simulink model "ES209A_CurrMeasCorrln"  (R2013b)
settings: Solver=FixedStepDiscrete  SolverMode=SingleTasking  StartTime=0.0  StopTime=1  FixedStep=0.000125  RelTol=1e-3
values from neighbouring files (symbols this model uses):
  CurrMeasCorrlnMaxErrCurr = DataDict.Calibration    [ES209A_CurrMeasCorrln_DataDict.m]
  CurrMeasCorrlnMaxStallCntr = DataDict.Calibration    [ES209A_CurrMeasCorrln_DataDict.m]
  CurrMeasCorrlnNtc0x04DFailStep = DataDict.Calibration    [ES209A_CurrMeasCorrln_DataDict.m]
  CurrMeasCorrlnNtc0x04DPassStep = DataDict.Calibration    [ES209A_CurrMeasCorrln_DataDict.m]
  CurrMeasCorrlnNtc0x04EFailStep = DataDict.Calibration    [ES209A_CurrMeasCorrln_DataDict.m]
  CurrMeasCorrlnNtc0x04EPassStep = DataDict.Calibration    [ES209A_CurrMeasCorrln_DataDict.m]
  ELECGLBPRM_IVTRCNT_CNT_U08 = DataDict.ConfigParam    [ES209A_CurrMeasCorrln_DataDict.m]
  FLTINJ_CURRMEASCORRLN_CURRMEASIDPTSIG = DataDict.Constant    [ES209A_CurrMeasCorrln_DataDict.m]
libraries: NxtrLim x2, simulink x1
(part 2 of 2)

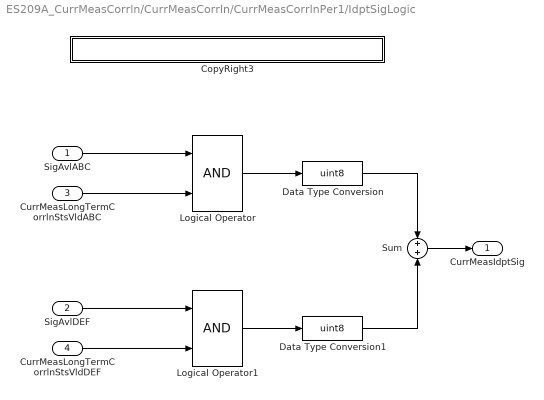
== system ES209A_CurrMeasCorrln/CurrMeasCorrln/CurrMeasCorrlnPer1/IdptSigLogic ==
  SigAvlABC : Inport  RequirementInfo={'linktype_rmi_doors' '0000c46e (/ESG Group/FDD Module Requirements/EA4 Specific/ES209A_CurrMeasCorrln)' '#ES209A_217' 'true' 'REQ: ES209A_217' '' ; 'linktype_rmi_doors' '0000c46e (/ESG Group/FDD Module Requirements/EA4 Specific/ES209A_CurrMeasCorrln)' '#ES209A_228' 'true' 'REQ: ES209A_228' '' ; 'linktype_rmi_doors' '0000c46e (/ESG Group/FDD Module Requirements/EA4 Specific/ES209A_CurrMeasCorrln)' '#ES209A_230' 'true' 'REQ: ES209A_230' '' ; 'linktype_rmi_doors' '0000c46e (/ESG Group/FDD Module Requirements/EA4 Specific/ES209A_CurrMeasCorrln)' '#ES209A_229' 'true' 'REQ: ES209A_229' '' } %GIDa_942e1c7b_ad02_468a_aa2a_044d99b82600
  SigAvlDEF : Inport  RequirementInfo={'linktype_rmi_doors' '0000c46e (/ESG Group/FDD Module Requirements/EA4 Specific/ES209A_CurrMeasCorrln)' '#ES209A_217' 'true' 'REQ: ES209A_217' '' ; 'linktype_rmi_doors' '0000c46e (/ESG Group/FDD Module Requirements/EA4 Specific/ES209A_CurrMeasCorrln)' '#ES209A_228' 'true' 'REQ: ES209A_228' '' ; 'linktype_rmi_doors' '0000c46e (/ESG Group/FDD Module Requirements/EA4 Specific/ES209A_CurrMeasCorrln)' '#ES209A_230' 'true' 'REQ: ES209A_230' '' ; 'linktype_rmi_doors' '0000c46e (/ESG Group/FDD Module Requirements/EA4 Specific/ES209A_CurrMeasCorrln)' '#ES209A_229' 'true' 'REQ: ES209A_229' '' } %GIDa_d76c2ed2_628a_4e52_8d10_5cc2fe66b57a  Port=2
  CurrMeasLongTermCorrlnStsVldABC : Inport  RequirementInfo={'linktype_rmi_doors' '0000c46e (/ESG Group/FDD Module Requirements/EA4 Specific/ES209A_CurrMeasCorrln)' '#ES209A_217' 'true' 'REQ: ES209A_217' '' ; 'linktype_rmi_doors' '0000c46e (/ESG Group/FDD Module Requirements/EA4 Specific/ES209A_CurrMeasCorrln)' '#ES209A_228' 'true' 'REQ: ES209A_228' '' ; 'linktype_rmi_doors' '0000c46e (/ESG Group/FDD Module Requirements/EA4 Specific/ES209A_CurrMeasCorrln)' '#ES209A_230' 'true' 'REQ: ES209A_230' '' ; 'linktype_rmi_doors' '0000c46e (/ESG Group/FDD Module Requirements/EA4 Specific/ES209A_CurrMeasCorrln)' '#ES209A_229' 'true' 'REQ: ES209A_229' '' } %GIDa_55133441_4ac9_4891_99c3_8d3056d5d792  Port=3
  CurrMeasLongTermCorrlnStsVldDEF : Inport  RequirementInfo={'linktype_rmi_doors' '0000c46e (/ESG Group/FDD Module Requirements/EA4 Specific/ES209A_CurrMeasCorrln)' '#ES209A_217' 'true' 'REQ: ES209A_217' '' ; 'linktype_rmi_doors' '0000c46e (/ESG Group/FDD Module Requirements/EA4 Specific/ES209A_CurrMeasCorrln)' '#ES209A_228' 'true' 'REQ: ES209A_228' '' ; 'linktype_rmi_doors' '0000c46e (/ESG Group/FDD Module Requirements/EA4 Specific/ES209A_CurrMeasCorrln)' '#ES209A_230' 'true' 'REQ: ES209A_230' '' ; 'linktype_rmi_doors' '0000c46e (/ESG Group/FDD Module Requirements/EA4 Specific/ES209A_CurrMeasCorrln)' '#ES209A_229' 'true' 'REQ: ES209A_229' '' } %GIDa_bf3bd0c8_6e6b_4ddf_a539_8fba819f64a3  Port=4
  CopyRight3 : Subsystem  Description=|  mask(Copyright Information){none=on}
      | Copyright info block.                                               
      |                                                                     
      | Place copyright information at the top of every subsystem in design.
      mask prompts: none "No parameters"
      mask help: Place copyright information at the top of every subsystem in design.
      mask Display:
      | NxtrConf = 'Nexteer Confidential';
      | 
      | sys = bdroot; %handle for the current model ("system")
      | first = get_param(sys,'Created');
      | first = first(end-3:end);  %year is last four digits
      | 
      | last = get_param(sys,'LastModifiedDate');
      | if isempty(last)
      |     last = datestr(now,'yyyy');
      | else
      |     last = last(end-3:end);
      | end
      | 
      | if strcmp(first,last)
      |     fprintf('%s -- Copyright %s Nexteer',NxtrConf,first)
      | else
      |     fprintf('%s -- %s%s- %s Nexteer',NxtrConf,char(169),first,last)
      | end
  Data Type Conversion : DataTypeConversion  RequirementInfo={'linktype_rmi_doors' '0000c46e (/ESG Group/FDD Module Requirements/EA4 Specific/ES209A_CurrMeasCorrln)' '#ES209A_217' 'true' 'REQ: ES209A_217' '' ; 'linktype_rmi_doors' '0000c46e (/ESG Group/FDD Module Requirements/EA4 Specific/ES209A_CurrMeasCorrln)' '#ES209A_228' 'true' 'REQ: ES209A_228' '' ; 'linktype_rmi_doors' '0000c46e (/ESG Group/FDD Module Requirements/EA4 Specific/ES209A_CurrMeasCorrln)' '#ES209A_230' 'true' 'REQ: ES209A_230' '' ; 'linktype_rmi_doors' '0000c46e (/ESG Group/FDD Module Requirements/EA4 Specific/ES209A_CurrMeasCorrln)' '#ES209A_229' 'true' 'REQ: ES209A_229' '' } %GIDa_5ccb0532_ac29_46e4_aa67_eafed2953408  OutDataTypeStr=uint8
  Data Type Conversion1 : DataTypeConversion  RequirementInfo={'linktype_rmi_doors' '0000c46e (/ESG Group/FDD Module Requirements/EA4 Specific/ES209A_CurrMeasCorrln)' '#ES209A_217' 'true' 'REQ: ES209A_217' '' ; 'linktype_rmi_doors' '0000c46e (/ESG Group/FDD Module Requirements/EA4 Specific/ES209A_CurrMeasCorrln)' '#ES209A_228' 'true' 'REQ: ES209A_228' '' ; 'linktype_rmi_doors' '0000c46e (/ESG Group/FDD Module Requirements/EA4 Specific/ES209A_CurrMeasCorrln)' '#ES209A_230' 'true' 'REQ: ES209A_230' '' ; 'linktype_rmi_doors' '0000c46e (/ESG Group/FDD Module Requirements/EA4 Specific/ES209A_CurrMeasCorrln)' '#ES209A_229' 'true' 'REQ: ES209A_229' '' } %GIDa_14c0623b_5dcd_41aa_bf12_39046edbd1db  OutDataTypeStr=uint8
  Logical Operator : Logic  RequirementInfo={'linktype_rmi_doors' '0000c46e (/ESG Group/FDD Module Requirements/EA4 Specific/ES209A_CurrMeasCorrln)' '#ES209A_217' 'true' 'REQ: ES209A_217' '' ; 'linktype_rmi_doors' '0000c46e (/ESG Group/FDD Module Requirements/EA4 Specific/ES209A_CurrMeasCorrln)' '#ES209A_228' 'true' 'REQ: ES209A_228' '' ; 'linktype_rmi_doors' '0000c46e (/ESG Group/FDD Module Requirements/EA4 Specific/ES209A_CurrMeasCorrln)' '#ES209A_230' 'true' 'REQ: ES209A_230' '' ; 'linktype_rmi_doors' '0000c46e (/ESG Group/FDD Module Requirements/EA4 Specific/ES209A_CurrMeasCorrln)' '#ES209A_229' 'true' 'REQ: ES209A_229' '' } %GIDa_2d1d910d_56b5_4346_ba27_43432a5aa696  IconShape=distinctive  AllPortsSameDT=off  OutDataTypeStr=boolean
  Logical Operator1 : Logic  RequirementInfo={'linktype_rmi_doors' '0000c46e (/ESG Group/FDD Module Requirements/EA4 Specific/ES209A_CurrMeasCorrln)' '#ES209A_217' 'true' 'REQ: ES209A_217' '' ; 'linktype_rmi_doors' '0000c46e (/ESG Group/FDD Module Requirements/EA4 Specific/ES209A_CurrMeasCorrln)' '#ES209A_228' 'true' 'REQ: ES209A_228' '' ; 'linktype_rmi_doors' '0000c46e (/ESG Group/FDD Module Requirements/EA4 Specific/ES209A_CurrMeasCorrln)' '#ES209A_230' 'true' 'REQ: ES209A_230' '' ; 'linktype_rmi_doors' '0000c46e (/ESG Group/FDD Module Requirements/EA4 Specific/ES209A_CurrMeasCorrln)' '#ES209A_229' 'true' 'REQ: ES209A_229' '' } %GIDa_f9654050_ad02_4c8d_9892_cac1300cf1d7  IconShape=distinctive  AllPortsSameDT=off  OutDataTypeStr=boolean
  Sum : Sum  RequirementInfo={'linktype_rmi_doors' '0000c46e (/ESG Group/FDD Module Requirements/EA4 Specific/ES209A_CurrMeasCorrln)' '#ES209A_217' 'true' 'REQ: ES209A_217' '' ; 'linktype_rmi_doors' '0000c46e (/ESG Group/FDD Module Requirements/EA4 Specific/ES209A_CurrMeasCorrln)' '#ES209A_228' 'true' 'REQ: ES209A_228' '' ; 'linktype_rmi_doors' '0000c46e (/ESG Group/FDD Module Requirements/EA4 Specific/ES209A_CurrMeasCorrln)' '#ES209A_230' 'true' 'REQ: ES209A_230' '' ; 'linktype_rmi_doors' '0000c46e (/ESG Group/FDD Module Requirements/EA4 Specific/ES209A_CurrMeasCorrln)' '#ES209A_229' 'true' 'REQ: ES209A_229' '' } %GIDa_4ade3bee_f5e6_4a94_82c8_89a81567cdbe  Inputs=+|+
  CurrMeasIdptSig : Outport  RequirementInfo={'linktype_rmi_doors' '0000c46e (/ESG Group/FDD Module Requirements/EA4 Specific/ES209A_CurrMeasCorrln)' '#ES209A_217' 'true' 'REQ: ES209A_217' '' ; 'linktype_rmi_doors' '0000c46e (/ESG Group/FDD Module Requirements/EA4 Specific/ES209A_CurrMeasCorrln)' '#ES209A_228' 'true' 'REQ: ES209A_228' '' ; 'linktype_rmi_doors' '0000c46e (/ESG Group/FDD Module Requirements/EA4 Specific/ES209A_CurrMeasCorrln)' '#ES209A_230' 'true' 'REQ: ES209A_230' '' ; 'linktype_rmi_doors' '0000c46e (/ESG Group/FDD Module Requirements/EA4 Specific/ES209A_CurrMeasCorrln)' '#ES209A_229' 'true' 'REQ: ES209A_229' '' } %GIDa_242059a7_1f05_43ee_b251_027ca547b730
  wires:
  SigAvlABC/1 -> Logical Operator/1
  CurrMeasLongTermCorrlnStsVldABC/1 -> Logical Operator/2
  CurrMeasLongTermCorrlnStsVldDEF/1 -> Logical Operator1/2
  SigAvlDEF/1 -> Logical Operator1/1
  Logical Operator/1 -> Data Type Conversion/1
  Logical Operator1/1 -> Data Type Conversion1/1
  Data Type Conversion/1 -> Sum/1
  Data Type Conversion1/1 -> Sum/2
  Sum/1 -> CurrMeasIdptSig/1

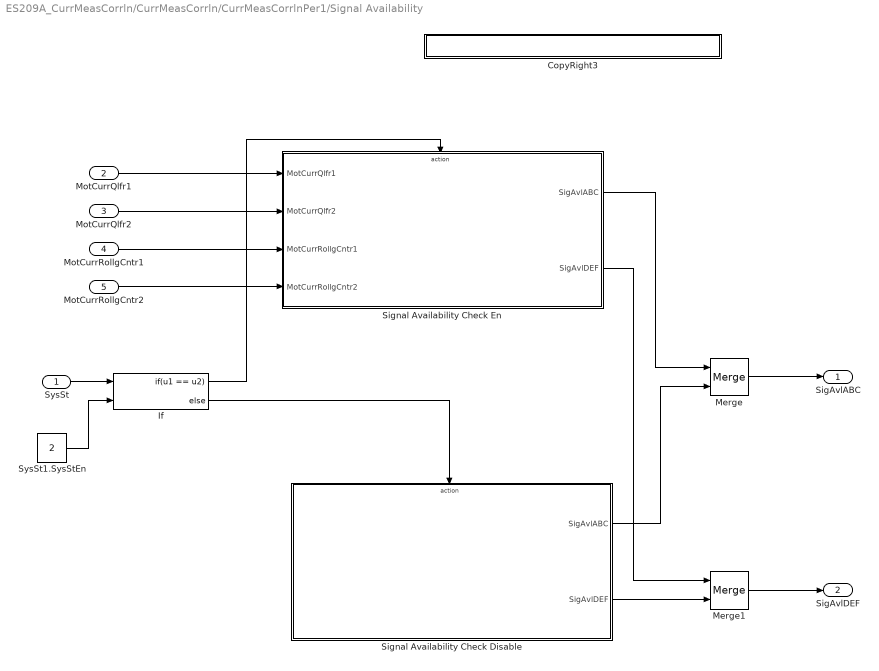
== system ES209A_CurrMeasCorrln/CurrMeasCorrln/CurrMeasCorrlnPer1/Signal Availability ==
  SysSt : Inport  RequirementInfo={} %GIDa_1186099d_dc67_4f7c_b378_ee59f8c97963  OutDataTypeStr=uint8
  MotCurrQlfr1 : Inport  RequirementInfo={} %GIDa_9546d9ec_22e7_463e_bbd0_54a2b6352662  Port=2
  MotCurrQlfr2 : Inport  RequirementInfo={} %GIDa_d3dc025e_ce3e_43df_848d_21e84192c51e  Port=3
  MotCurrRollgCntr1 : Inport  RequirementInfo={} %GIDa_8e4ee91b_32ff_41c2_995e_2ae76632680d  Port=4
  MotCurrRollgCntr2 : Inport  RequirementInfo={} %GIDa_46b1cb0c_dece_4346_b2ac_908178a65c66  Port=5
  CopyRight3 : Subsystem  Description=|  mask(Copyright Information){none=on}
      | Copyright info block.                                               
      |                                                                     
      | Place copyright information at the top of every subsystem in design.
      mask prompts: none "No parameters"
      mask help: Place copyright information at the top of every subsystem in design.
      mask Display:
      | NxtrConf = 'Nexteer Confidential';
      | 
      | sys = bdroot; %handle for the current model ("system")
      | first = get_param(sys,'Created');
      | first = first(end-3:end);  %year is last four digits
      | 
      | last = get_param(sys,'LastModifiedDate');
      | if isempty(last)
      |     last = datestr(now,'yyyy');
      | else
      |     last = last(end-3:end);
      | end
      | 
      | if strcmp(first,last)
      |     fprintf('%s -- Copyright %s Nexteer',NxtrConf,first)
      | else
      |     fprintf('%s -- %s%s- %s Nexteer',NxtrConf,char(169),first,last)
      | end
  If : If  NumInputs=2  IfExpression=u1 == u2
  Merge : Merge
  Merge1 : Merge
  Signal Availability Check Disable : Subsystem  RequirementInfo={} %GIDa_6318f0e3_a9ed_4028_939a_acdca8fc9a22  TreatAsAtomicUnit=on
  Signal Availability Check En : Subsystem  RequirementInfo={'linktype_rmi_doors' '0000c46e (/ESG Group/FDD Module Requirements/EA4 Specific/ES209A CurrMeasCorrln)' '#ES209A_135' 'true' 'REQ: ES209A_135' '' } %GIDa_7e57cf61_2110_43cd_98fc_69fb451c1a76  TreatAsAtomicUnit=on
  SysSt1.SysStEn : Constant  Value=2  OutDataTypeStr=uint8
  SigAvlABC : Outport
  SigAvlDEF : Outport  Port=2
  wires:
  SysSt/1 -> If/1
  SysSt1.SysStEn/1 -> If/2
  MotCurrQlfr1/1 -> Signal Availability Check En/1(MotCurrQlfr1)
  MotCurrQlfr2/1 -> Signal Availability Check En/2(MotCurrQlfr2)
  MotCurrRollgCntr1/1 -> Signal Availability Check En/3(MotCurrRollgCntr1)
  MotCurrRollgCntr2/1 -> Signal Availability Check En/4(MotCurrRollgCntr2)
  Signal Availability Check En/1(SigAvlABC) -> Merge/1
  Signal Availability Check Disable/1(SigAvlABC) -> Merge/2
  Signal Availability Check En/2("SigAvlDEF ") -> Merge1/1
  Signal Availability Check Disable/2("SigAvlDEF ") -> Merge1/2
  Merge/1 -> SigAvlABC/1
  Merge1/1 -> SigAvlDEF/1
  If/2 -> Signal Availability Check Disable/Action
  If/1 -> Signal Availability Check En/Action

== system ES209A_CurrMeasCorrln/CurrMeasCorrln/CurrMeasCorrlnPer1/CorrlnChkABC/GetNtcQlfrSts/CopyRight2 ==

== system ES209A_CurrMeasCorrln/CurrMeasCorrln/CurrMeasCorrlnPer1/CorrlnChkABC/ImdtCorrlnCk/CopyRight2 ==

== system ES209A_CurrMeasCorrln/CurrMeasCorrln/CurrMeasCorrlnPer1/CorrlnChkABC/ImdtCorrlnCk/If Action Subsystem ==
  Action Port : ActionPort  ActionType=then
  Constant : Constant
  ImdtCorrlnABC : Outport
  wires:
  Constant/1 -> ImdtCorrlnABC/1

== system ES209A_CurrMeasCorrln/CurrMeasCorrln/CurrMeasCorrlnPer1/CorrlnChkABC/ImdtCorrlnCk/If Action Subsystem1 ==
  Action Port : ActionPort  ActionType=else
  Constant : Constant  Value=0
  ImdtCorrlnABC : Outport
  wires:
  Constant/1 -> ImdtCorrlnABC/1

== system ES209A_CurrMeasCorrln/CurrMeasCorrln/CurrMeasCorrlnPer1/CorrlnChkABC/SetNtcSts/CopyRight2 ==

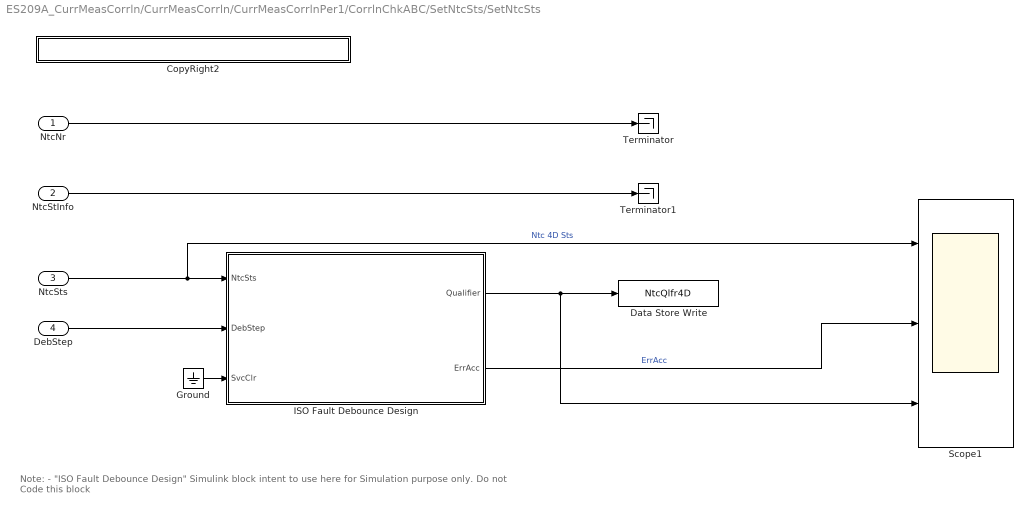
== system ES209A_CurrMeasCorrln/CurrMeasCorrln/CurrMeasCorrlnPer1/CorrlnChkABC/SetNtcSts/SetNtcSts ==
  note: Note:
      |
      | - "ISO Fault Debounce Design" Simulink block intent to use here for Simulation purpose only. Do not Code this block
  NtcNr : Inport
  NtcStInfo : Inport  Port=2
  NtcSts : Inport  Port=3
  DebStep : Inport  Port=4
  CopyRight2 : Subsystem  Description=|  mask(Copyright Information){none=on}
      | Copyright info block.                                               
      |                                                                     
      | Place copyright information at the top of every subsystem in design.
      mask prompts: none "No parameters"
      mask help: Place copyright information at the top of every subsystem in design.
      mask Display:
      | NxtrConf = 'Nexteer Confidential';
      | 
      | sys = bdroot; %handle for the current model ("system")
      | first = get_param(sys,'Created');
      | first = first(end-3:end);  %year is last four digits
      | 
      | last = get_param(sys,'LastModifiedDate');
      | if isempty(last)
      |     last = datestr(now,'yyyy');
      | else
      |     last = last(end-3:end);
      | end
      | 
      | if strcmp(first,last)
      |     fprintf('%s -- Copyright %s Nexteer',NxtrConf,first)
      | else
      |     fprintf('%s -- %s%s- %s Nexteer',NxtrConf,char(169),first,last)
      | end
  Data Store Write : DataStoreWrite  DataStoreName=NtcQlfr4D
  Ground : Ground
  ISO Fault Debounce Design : Stateflow chart  RequirementInfo={'linktype_rmi_doors' '0000c46e (/ESG Group/FDD Module Requirements/EA4 Specific/ES209A CurrMeasCorrln)' '#ES209A_236' 'true' 'REQ: ES209A_236' '' } %GIDa_d30caf31_34ad_4c46_80cc_2f0c0a5a5e0e  TreatAsAtomicUnit=on
      settings: AttributesFormatString=|
      | Simulation Purpose Only.
      | Do Not Code this block
      | Diagnostic Manager Owns this requirement
  Scope1 : Scope  NumInputPorts=3
      settings: YMin=2~-35000~0  YMax=3~35000~1  SaveName=ScopeData4
  Terminator : Terminator
  Terminator1 : Terminator
  wires:
  NtcStInfo/1 -> Terminator1/1
  NtcNr/1 -> Terminator/1
  DebStep/1 -> ISO Fault Debounce Design/2(DebStep)
  ISO Fault Debounce Design/1(Qualifier) -> Scope1/3, Data Store Write/1
  Ground/1 -> ISO Fault Debounce Design/3(SvcClr)
  ISO Fault Debounce Design/2(ErrAcc) -> Scope1/2  "ErrAcc"
  NtcSts/1 -> Scope1/1, ISO Fault Debounce Design/1(NtcSts)  "Ntc 4D Sts"

== system ES209A_CurrMeasCorrln/CurrMeasCorrln/CurrMeasCorrlnPer1/CorrlnChkDEF/GetNtcQlfrSts/CopyRight2 ==

== system ES209A_CurrMeasCorrln/CurrMeasCorrln/CurrMeasCorrlnPer1/CorrlnChkDEF/ImdtCorrlnCk/CopyRight2 ==

== system ES209A_CurrMeasCorrln/CurrMeasCorrln/CurrMeasCorrlnPer1/CorrlnChkDEF/ImdtCorrlnCk/If Action Subsystem ==
  Action Port : ActionPort  ActionType=then
  Constant : Constant
  ImdtCorrlnABC : Outport
  wires:
  Constant/1 -> ImdtCorrlnABC/1

== system ES209A_CurrMeasCorrln/CurrMeasCorrln/CurrMeasCorrlnPer1/CorrlnChkDEF/ImdtCorrlnCk/If Action Subsystem1 ==
  Action Port : ActionPort  ActionType=else
  Constant : Constant  Value=0
  ImdtCorrlnABC : Outport
  wires:
  Constant/1 -> ImdtCorrlnABC/1

== system ES209A_CurrMeasCorrln/CurrMeasCorrln/CurrMeasCorrlnPer1/CorrlnChkDEF/SetNtcSts/CopyRight2 ==

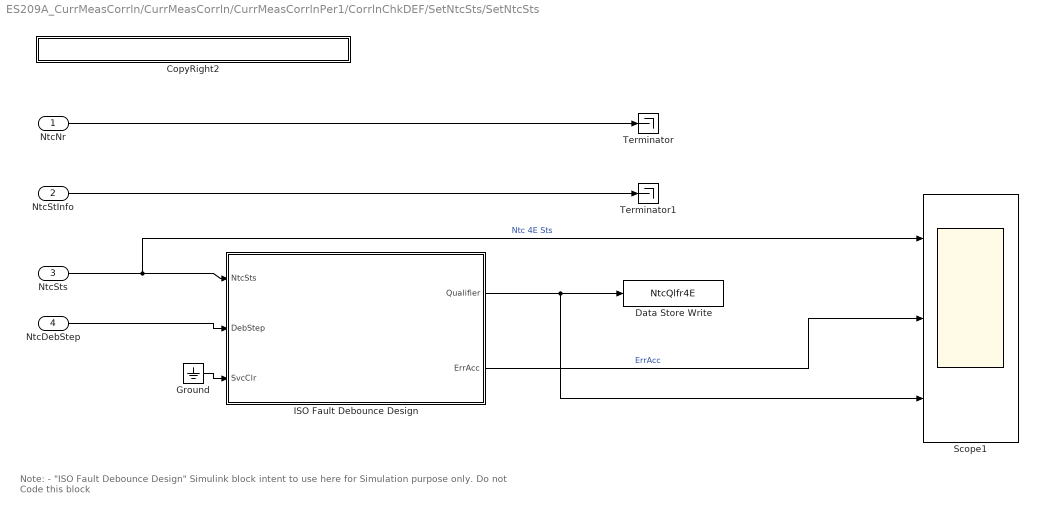
== system ES209A_CurrMeasCorrln/CurrMeasCorrln/CurrMeasCorrlnPer1/CorrlnChkDEF/SetNtcSts/SetNtcSts ==
  note: Note:
      |
      | - "ISO Fault Debounce Design" Simulink block intent to use here for Simulation purpose only. Do not Code this block
  NtcNr : Inport
  NtcStInfo : Inport  Port=2
  NtcSts : Inport  Port=3
  NtcDebStep : Inport  Port=4
  CopyRight2 : Subsystem  Description=|  mask(Copyright Information){none=on}
      | Copyright info block.                                               
      |                                                                     
      | Place copyright information at the top of every subsystem in design.
      mask prompts: none "No parameters"
      mask help: Place copyright information at the top of every subsystem in design.
      mask Display:
      | NxtrConf = 'Nexteer Confidential';
      | 
      | sys = bdroot; %handle for the current model ("system")
      | first = get_param(sys,'Created');
      | first = first(end-3:end);  %year is last four digits
      | 
      | last = get_param(sys,'LastModifiedDate');
      | if isempty(last)
      |     last = datestr(now,'yyyy');
      | else
      |     last = last(end-3:end);
      | end
      | 
      | if strcmp(first,last)
      |     fprintf('%s -- Copyright %s Nexteer',NxtrConf,first)
      | else
      |     fprintf('%s -- %s%s- %s Nexteer',NxtrConf,char(169),first,last)
      | end
  Data Store Write : DataStoreWrite  DataStoreName=NtcQlfr4E
  Ground : Ground
  ISO Fault Debounce Design : Stateflow chart  RequirementInfo={'linktype_rmi_doors' '0000c46e (/ESG Group/FDD Module Requirements/EA4 Specific/ES209A CurrMeasCorrln)' '#ES209A_252' 'true' 'REQ: ES209A_252' '' } %GIDa_7a5c8c14_f745_4195_88a1_5e88b55f3450  TreatAsAtomicUnit=on
      settings: AttributesFormatString=|
      | Simulation Purpose Only.
      | Do Not Code this block
      | Diagnostic Manager Owns this requirement
  Scope1 : Scope  NumInputPorts=3
      settings: YMin=2~-35000~0  YMax=3~35000~2  SaveName=ScopeData4
  Terminator : Terminator
  Terminator1 : Terminator
  wires:
  NtcStInfo/1 -> Terminator1/1
  NtcNr/1 -> Terminator/1
  NtcSts/1 -> ISO Fault Debounce Design/1(NtcSts), Scope1/1  "Ntc 4E Sts"
  NtcDebStep/1 -> ISO Fault Debounce Design/2(DebStep)
  ISO Fault Debounce Design/1(Qualifier) -> Scope1/3, Data Store Write/1
  Ground/1 -> ISO Fault Debounce Design/3(SvcClr)
  ISO Fault Debounce Design/2(ErrAcc) -> Scope1/2  "ErrAcc"

== system ES209A_CurrMeasCorrln/CurrMeasCorrln/CurrMeasCorrlnPer1/CorrlnStsLogic/CopyRight3 ==

== system ES209A_CurrMeasCorrln/CurrMeasCorrln/CurrMeasCorrlnPer1/FltInj_u08/CopyRight1 ==

== system ES209A_CurrMeasCorrln/CurrMeasCorrln/CurrMeasCorrlnPer1/IdptSigLogic/CopyRight3 ==

== system ES209A_CurrMeasCorrln/CurrMeasCorrln/CurrMeasCorrlnPer1/Signal Availability/CopyRight3 ==

== system ES209A_CurrMeasCorrln/CurrMeasCorrln/CurrMeasCorrlnPer1/Signal Availability/Signal Availability Check Disable ==
  Action Port : ActionPort  ActionType=else
  Constant : Constant  OutDataTypeStr=uint8
  Constant1 : Constant  OutDataTypeStr=uint8
  CopyRight3 : Subsystem  Description=|  mask(Copyright Information){none=on}
      | Copyright info block.                                               
      |                                                                     
      | Place copyright information at the top of every subsystem in design.
      mask prompts: none "No parameters"
      mask help: Place copyright information at the top of every subsystem in design.
      mask Display:
      | NxtrConf = 'Nexteer Confidential';
      | 
      | sys = bdroot; %handle for the current model ("system")
      | first = get_param(sys,'Created');
      | first = first(end-3:end);  %year is last four digits
      | 
      | last = get_param(sys,'LastModifiedDate');
      | if isempty(last)
      |     last = datestr(now,'yyyy');
      | else
      |     last = last(end-3:end);
      | end
      | 
      | if strcmp(first,last)
      |     fprintf('%s -- Copyright %s Nexteer',NxtrConf,first)
      | else
      |     fprintf('%s -- %s%s- %s Nexteer',NxtrConf,char(169),first,last)
      | end
  SigAvlABC : Outport
  "SigAvlDEF " : Outport  Port=2
  wires:
  Constant1/1 -> "SigAvlDEF "/1
  Constant/1 -> SigAvlABC/1

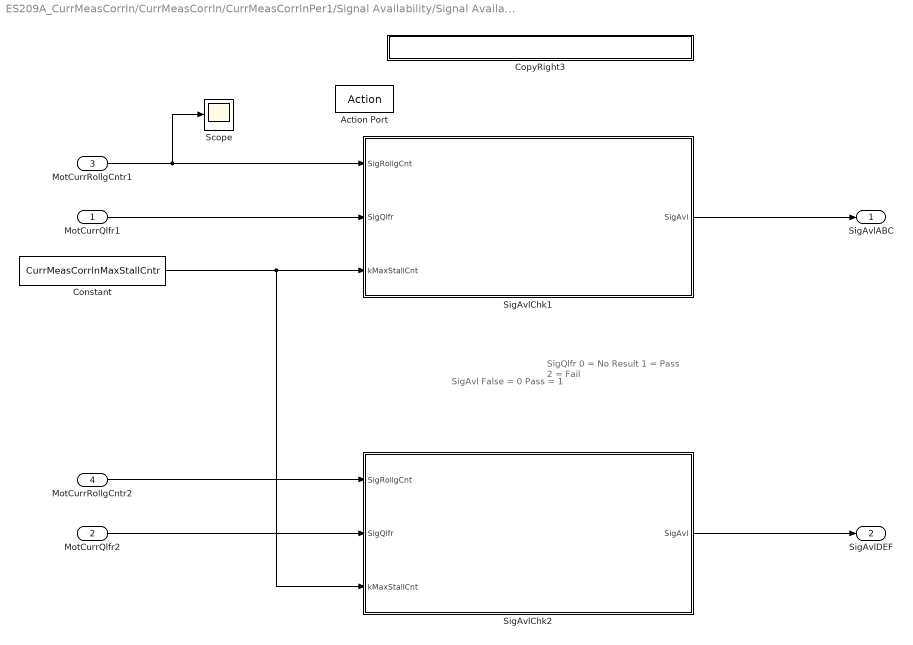
== system ES209A_CurrMeasCorrln/CurrMeasCorrln/CurrMeasCorrlnPer1/Signal Availability/Signal Availability Check En ==
  note: SigQlfr
      | 0 = No Result
      | 1 = Pass
      | 2 = Fail
  note: SigAvl
      | False = 0
      | Pass = 1
  MotCurrQlfr1 : Inport  RequirementInfo={} %GIDa_023689e3_7c9e_4df1_83a1_699197148238
  MotCurrQlfr2 : Inport  RequirementInfo={} %GIDa_7e6e4398_831d_4c26_91b8_cbf4c078805f  Port=2
  MotCurrRollgCntr1 : Inport  RequirementInfo={} %GIDa_382efb02_9c14_4780_8bc5_4a8377343de5  Port=3
  MotCurrRollgCntr2 : Inport  RequirementInfo={} %GIDa_533c6f48_88f4_4233_bfc1_2f844aa0d431  Port=4
  Action Port : ActionPort  ActionType=then
  Constant : Constant  Value=CurrMeasCorrlnMaxStallCntr
  CopyRight3 : Subsystem  Description=|  mask(Copyright Information){none=on}
      | Copyright info block.                                               
      |                                                                     
      | Place copyright information at the top of every subsystem in design.
      mask prompts: none "No parameters"
      mask help: Place copyright information at the top of every subsystem in design.
      mask Display:
      | NxtrConf = 'Nexteer Confidential';
      | 
      | sys = bdroot; %handle for the current model ("system")
      | first = get_param(sys,'Created');
      | first = first(end-3:end);  %year is last four digits
      | 
      | last = get_param(sys,'LastModifiedDate');
      | if isempty(last)
      |     last = datestr(now,'yyyy');
      | else
      |     last = last(end-3:end);
      | end
      | 
      | if strcmp(first,last)
      |     fprintf('%s -- Copyright %s Nexteer',NxtrConf,first)
      | else
      |     fprintf('%s -- %s%s- %s Nexteer',NxtrConf,char(169),first,last)
      | end
  Scope : Scope
  SigAvlChk1 : Subsystem  RequirementInfo={'linktype_rmi_doors' '0000c46e (/ESG Group/FDD Module Requirements/EA4 Specific/ES209A CurrMeasCorrln)' '#ES209A_135' 'true' 'REQ: ES209A_135' '' } %GIDa_5a6e0e53_d246_4b66_936c_563396a92aca  TreatAsAtomicUnit=on
  SigAvlChk2 : Subsystem  RequirementInfo={'linktype_rmi_doors' '0000c46e (/ESG Group/FDD Module Requirements/EA4 Specific/ES209A CurrMeasCorrln)' '#ES209A_219' 'true' 'REQ: ES209A_219' '' } %GIDa_e73a73aa_ed9a_4202_a7ed_28e935db4abc  TreatAsAtomicUnit=on
  SigAvlABC : Outport
  "SigAvlDEF " : Outport  Port=2
  wires:
  MotCurrRollgCntr1/1 -> SigAvlChk1/1(SigRollgCnt), Scope/1
  MotCurrQlfr1/1 -> SigAvlChk1/2(SigQlfr)
  MotCurrRollgCntr2/1 -> SigAvlChk2/1(SigRollgCnt)
  MotCurrQlfr2/1 -> SigAvlChk2/2(SigQlfr)
  Constant/1 -> SigAvlChk2/3(kMaxStallCnt), SigAvlChk1/3(kMaxStallCnt)
  SigAvlChk2/1(SigAvl) -> "SigAvlDEF "/1
  SigAvlChk1/1(SigAvl) -> SigAvlABC/1

== system ES209A_CurrMeasCorrln/CurrMeasCorrln/CurrMeasCorrlnPer1/CorrlnChkABC/SetNtcSts/SetNtcSts/CopyRight2 ==

== system ES209A_CurrMeasCorrln/CurrMeasCorrln/CurrMeasCorrlnPer1/CorrlnChkDEF/SetNtcSts/SetNtcSts/CopyRight2 ==

== system ES209A_CurrMeasCorrln/CurrMeasCorrln/CurrMeasCorrlnPer1/Signal Availability/Signal Availability Check Disable/CopyRight3 ==

== system ES209A_CurrMeasCorrln/CurrMeasCorrln/CurrMeasCorrlnPer1/Signal Availability/Signal Availability Check En/CopyRight3 ==

== system ES209A_CurrMeasCorrln/CurrMeasCorrln/CurrMeasCorrlnPer1/Signal Availability/Signal Availability Check En/SigAvlChk1 ==
  note: Example of PIM declaration for StallCnt State Variable
      |
      | SnsrShoNameSens0StallCntPrev = DataDict.PIM;
      | SnsrShoNameSens0StallCntPrev.LongName = 'SnsrShoNameSens0RollgCntPrev';
      | SnsrShoNameSens0StallCntPrev.Description = 'SnsrShoNameSens0RollgCntPrev';
      | SnsrShoNameSens0StallCntPrev.DocUnits = 'Cnt';
      | SnsrShoNameSens0StallCntPrev.EngDT = dt.u08;
      | SnsrShoNameSens0StallCntPrev.EngInit = 0;
      | SnsrShoNameSens0StallCntPrev.EngMin = 0;
      | SnsrShoNameSens0StallCntPrev.EngMax = 255;
      |
      |
      | *********  Need different state variable for each instance of this  subsystem ********
  note: Example of PIM declaration for RollgCnt State Variable
      |
      | SnsrShoNameSens0RollgCntPrev = DataDict.PIM;
      | SnsrShoNameSens0RollgCntPrev.LongName = 'SnsrShoNameSens0RollgCntPrev';
      | SnsrShoNameSens0RollgCntPrev.Description = 'SnsrShoNameSens0RollgCntPrev';
      | SnsrShoNameSens0RollgCntPrev.DocUnits = 'Cnt';
      | SnsrShoNameSens0RollgCntPrev.EngDT = dt.u08;
      | SnsrShoNameSens0RollgCntPrev.EngInit = 0;
      | SnsrShoNameSens0RollgCntPrev.EngMin = 0;
      | SnsrShoNameSens0RollgCntPrev.EngMax = 255;
      |
      |
      | *********  Need different state variable for each instance of this  subsystem ********
  SigRollgCnt : Inport  OutDataTypeStr=uint8
  SigQlfr : Inport  Port=2  OutDataTypeStr=uint8
  kMaxStallCnt : Inport  Port=3  OutDataTypeStr=uint8
  CopyRight1 : Subsystem  Description=|  mask(Copyright Information){none=on}
      | Copyright info block.                                               
      |                                                                     
      | Place copyright information at the top of every subsystem in design.
      mask prompts: none "No parameters"
      mask help: Place copyright information at the top of every subsystem in design.
      mask Display:
      | NxtrConf = 'Nexteer Confidential';
      | 
      | sys = bdroot; %handle for the current model ("system")
      | first = get_param(sys,'Created');
      | first = first(end-3:end);  %year is last four digits
      | 
      | last = get_param(sys,'LastModifiedDate');
      | if isempty(last)
      |     last = datestr(now,'yyyy');
      | else
      |     last = last(end-3:end);
      | end
      | 
      | if strcmp(first,last)
      |     fprintf('%s -- Copyright %s Nexteer',NxtrConf,first)
      | else
      |     fprintf('%s -- %s%s- %s Nexteer',NxtrConf,char(169),first,last)
      | end
  Display2 : Display
  Display3 : Display
  SigAvlChkRev2 : Stateflow chart  TreatAsAtomicUnit=on
  Unit Delay : UnitDelay  SampleTime=-1  StateName=Snsr0RollgCntPrev  StateMustResolveToSignalObject=on
      settings: AttributesFormatString=|
      | State Variable:
      | %<StateName>
  Unit Delay1 : UnitDelay  SampleTime=-1  StateName=Snsr0StallCntPrev  StateMustResolveToSignalObject=on
      settings: AttributesFormatString=|
      | State Variable:
      | %<StateName>
  SigAvl : Outport
  wires:
  SigRollgCnt/1 -> Unit Delay/1, Display2/1, SigAvlChkRev2/1(SigRollgCnt)  "SigRollgCnt"
  SigQlfr/1 -> Display3/1, SigAvlChkRev2/2(SigQlfr)  "SigQlfr"
  kMaxStallCnt/1 -> SigAvlChkRev2/3(kMaxStallCnt)  "kMaxStallCnt"
  Unit Delay/1 -> SigAvlChkRev2/4(LstRollgCnt)
  SigAvlChkRev2/2(StallCntOutp) -> Unit Delay1/1
  Unit Delay1/1 -> SigAvlChkRev2/5(LstStallCnt)
  SigAvlChkRev2/1(SigAvl) -> SigAvl/1

== system ES209A_CurrMeasCorrln/CurrMeasCorrln/CurrMeasCorrlnPer1/Signal Availability/Signal Availability Check En/SigAvlChk2 ==
  note: Example of PIM declaration for StallCnt State Variable
      |
      | SnsrShoNameSens0StallCntPrev = DataDict.PIM;
      | SnsrShoNameSens0StallCntPrev.LongName = 'SnsrShoNameSens0RollgCntPrev';
      | SnsrShoNameSens0StallCntPrev.Description = 'SnsrShoNameSens0RollgCntPrev';
      | SnsrShoNameSens0StallCntPrev.DocUnits = 'Cnt';
      | SnsrShoNameSens0StallCntPrev.EngDT = dt.u08;
      | SnsrShoNameSens0StallCntPrev.EngInit = 0;
      | SnsrShoNameSens0StallCntPrev.EngMin = 0;
      | SnsrShoNameSens0StallCntPrev.EngMax = 255;
      |
      |
      | *********  Need different state variable for each instance of this  subsystem ********
  note: Example of PIM declaration for RollgCnt State Variable
      |
      | SnsrShoNameSens0RollgCntPrev = DataDict.PIM;
      | SnsrShoNameSens0RollgCntPrev.LongName = 'SnsrShoNameSens0RollgCntPrev';
      | SnsrShoNameSens0RollgCntPrev.Description = 'SnsrShoNameSens0RollgCntPrev';
      | SnsrShoNameSens0RollgCntPrev.DocUnits = 'Cnt';
      | SnsrShoNameSens0RollgCntPrev.EngDT = dt.u08;
      | SnsrShoNameSens0RollgCntPrev.EngInit = 0;
      | SnsrShoNameSens0RollgCntPrev.EngMin = 0;
      | SnsrShoNameSens0RollgCntPrev.EngMax = 255;
      |
      |
      | *********  Need different state variable for each instance of this  subsystem ********
  SigRollgCnt : Inport  OutDataTypeStr=uint8
  SigQlfr : Inport  Port=2  OutDataTypeStr=uint8
  kMaxStallCnt : Inport  Port=3  OutDataTypeStr=uint8
  CopyRight2 : Subsystem  Description=|  mask(Copyright Information){none=on}
      | Copyright info block.                                               
      |                                                                     
      | Place copyright information at the top of every subsystem in design.
      mask prompts: none "No parameters"
      mask help: Place copyright information at the top of every subsystem in design.
      mask Display:
      | NxtrConf = 'Nexteer Confidential';
      | 
      | sys = bdroot; %handle for the current model ("system")
      | first = get_param(sys,'Created');
      | first = first(end-3:end);  %year is last four digits
      | 
      | last = get_param(sys,'LastModifiedDate');
      | if isempty(last)
      |     last = datestr(now,'yyyy');
      | else
      |     last = last(end-3:end);
      | end
      | 
      | if strcmp(first,last)
      |     fprintf('%s -- Copyright %s Nexteer',NxtrConf,first)
      | else
      |     fprintf('%s -- %s%s- %s Nexteer',NxtrConf,char(169),first,last)
      | end
  Display2 : Display
  Display3 : Display
  SigAvlChkRev2 : Stateflow chart  TreatAsAtomicUnit=on
  Unit Delay : UnitDelay  SampleTime=-1  StateName=Snsr1RollgCntPrev  StateMustResolveToSignalObject=on
      settings: AttributesFormatString=|
      | State Variable:
      | %<StateName>
  Unit Delay1 : UnitDelay  SampleTime=-1  StateName=Snsr1StallCntPrev  StateMustResolveToSignalObject=on
      settings: AttributesFormatString=|
      | State Variable:
      | %<StateName>
  SigAvl : Outport
  wires:
  SigRollgCnt/1 -> Unit Delay/1, Display2/1, SigAvlChkRev2/1(SigRollgCnt)  "SigRollgCnt"
  SigQlfr/1 -> Display3/1, SigAvlChkRev2/2(SigQlfr)  "SigQlfr"
  kMaxStallCnt/1 -> SigAvlChkRev2/3(kMaxStallCnt)  "kMaxStallCnt"
  Unit Delay/1 -> SigAvlChkRev2/4(LstRollgCnt)
  SigAvlChkRev2/2(StallCntOutp) -> Unit Delay1/1
  Unit Delay1/1 -> SigAvlChkRev2/5(LstStallCnt)
  SigAvlChkRev2/1(SigAvl) -> SigAvl/1

== system ES209A_CurrMeasCorrln/CurrMeasCorrln/CurrMeasCorrlnPer1/Signal Availability/Signal Availability Check En/SigAvlChk1/CopyRight1 ==

== system ES209A_CurrMeasCorrln/CurrMeasCorrln/CurrMeasCorrlnPer1/Signal Availability/Signal Availability Check En/SigAvlChk2/CopyRight2 ==

== stateflow chart ES209A_CurrMeasCorrln/CurrMeasCorrln/CurrMeasCorrlnPer1/CorrlnChkABC ==
  state [ImdtCorrlnABC,CurrMotSumABC] = ImdtCorrlnCk(MotCurrCorrdA,MotCurrCorrdB,MotCurrCorrdC) [function]
  note: /******************************
      | Change for 2.9.0
      | CurrMotSumABC = 0;
      | ******************************/
  state CurrMeasCorrlnNtcSet = SetNtcSts(NTCNr,ParamBit,NTCSts,NTCDebStep) [function]
  note: Rationale for CurrMotSumABC = 0:
      | This is notifying state of health that CurrMotSum
      | is OK when it is not evaluated.   Since state of health
      | latches the most "unhealthy" value of the signal
      | it has received, this will have no impact on state of health.
  state NtcQlfr1 = GetNtcQlfrSts(NtcNr) [function]
  (default) -> (junction 128)
  (junction 128) -> (junction 138) [order 2] : {CurrMeasImdtCorrlnStsVldABC = 1;
      | CurrMeasLongTermCorrlnStsVldABC = 1;
      | CurrMotSumABC = 0;}
  (junction 128) -> (junction 142) [order 1] : [SysSt == 2]
  (junction 142) -> (junction 138) [order 2] : {CurrMeasImdtCorrlnStsVldABC = 0;
      | CurrMeasLongTermCorrlnStsVldABC = 0;
      | CurrMotSumABC = 0;}
  (junction 142) -> (junction 53) [order 1] : [DiagcStsIvtr1Inactv == 0 && MotCurrEolCalSt == 0]
      |
      | {[ImdtCorrlnABC, CurrMotSumABC] = ImdtCorrlnCk(MotCurrCorrdA, MotCurrCorrdB, MotCurrCorrdC);}
  (junction 53) -> (junction 75) [order 2]
  (junction 53) -> (junction 57) [order 1] : [ImdtCorrlnABC == 1]
  (junction 57) -> (junction 89) : {CurrMeasImdtCorrlnStsVldABC = 1;
      | SetNtcSts(NTCNR_0X04D, 0, 2, CurrMeasCorrlnNtc0x04DPassStep);}
  (junction 75) -> (junction 90) : {CurrMeasImdtCorrlnStsVldABC = 0;
      | SetNtcSts(NTCNR_0X04D, 1, 3, CurrMeasCorrlnNtc0x04DFailStep);}
  (junction 89) -> (junction 93)
  (junction 90) -> (junction 93)
  (junction 93) -> (junction 102) : {CorrlnNtc4DQlfrSts = GetNtcQlfrSts(NTCNR_0X04D);}
  (junction 102) -> (junction 103) [order 1] : [CorrlnNtc4DQlfrSts == 2]
      | {CurrMeasLongTermCorrlnStsVldABC = 0;}
  (junction 102) -> (junction 103) [order 2] : {CurrMeasLongTermCorrlnStsVldABC = 1;}
  (junction 103) -> (junction 138)
  data: MotCurrCorrdA function_input double; MotCurrCorrdB function_input double; MotCurrCorrdC function_input double; ImdtCorrlnABC function_output; CurrMotSumABC function_output; NTCNr function_input; ParamBit function_input; CurrMeasCorrlnNtcSet function_output; NTCSts function_input; NTCDebStep function_input; NtcNr function_input; NtcQlfr1 function_output; MotCurrCorrdA input single; MotCurrCorrdB input single; MotCurrCorrdC input single; CurrMeasLongTermCorrlnNtc4DSet local uint8; CorrlnNtc4DQlfrSts local uint8; CurrMeasCorrlnNtc0x04DPassStep input; CurrMeasCorrlnNtc0x04DFailStep input; SysSt input; CurrMeasImdtCorrlnStsVldABC output uint8; CurrMeasLongTermCorrlnStsVldABC output uint8; NTCNR_0X04D constant uint16 =77; DiagcStsIvtr1Inactv input; MotCurrEolCalSt input; CurrMotSumABC output single; ImdtCorrlnABC local double

== stateflow chart ES209A_CurrMeasCorrln/CurrMeasCorrln/CurrMeasCorrlnPer1/CorrlnChkABC/SetNtcSts/SetNtcSts/ISO Fault Debounce Design ==
  note: Pass Loop
  note: Fail Loop
  note: 
  note: NTCSTS_PASSD           (0)
      | NTCSTS_FAILD             (1)
      | NTCSTS_PREPASSD   (2)
      | NTCSTS_PREFAILD     (3)
      |
      | SIGQLFR_NORES        (0)
      | SIGQLFR_PASSD         (1)
      | SIGQLFR_FAILD           (2)
  (default) -> (junction 89)
  (junction 89) -> (junction 95) [order 1] : [NtcSts ==3]
  (junction 89) -> (junction 93) [order 2] : [NtcSts ==2]
  (junction 89) -> (junction 141) [order 3] : [NtcSts ==1]
      | { ErrAcc = 32767;
      | Qualifier =2;
      |  }
  (junction 89) -> (junction 141) [order 4] : [NtcSts ==0]
      | { ErrAcc = -32768;
      | Qualifier=1;
      | }
  (junction 95) -> (junction 103) [order 2]
  (junction 95) -> (junction 111) [order 1] : [ErrAcc <=0]
      | {ErrAcc = DebStep;}
  (junction 93) -> (junction 123) [order 2] : {
      | ErrAcc = ErrAcc - DebStep;
      | }
  (junction 93) -> (junction 123) [order 1] : [(ErrAcc - DebStep) <= -32768]
      | { ErrAcc = -32768;
      | Qualifier=1;
      | }
  (junction 103) -> (junction 111) [order 1] : [(ErrAcc + DebStep) <32767]
      | {ErrAcc = ErrAcc + DebStep;}
  (junction 103) -> (junction 111) [order 2] : {ErrAcc = 32767;
      | Qualifier =2;}
  (junction 123) -> (junction 141)
  (junction 111) -> (junction 141)
  (junction 141) -> (junction 159) [order 1] : [SvcClr ==1]
      | {ErrAcc = 0;
      | Qualifier =0;
      | }
  (junction 141) -> (junction 159) [order 2]
  data: NtcSts input uint8; Qualifier output uint8; DebStep input int32; ErrAcc output single; SvcClr input

== stateflow chart ES209A_CurrMeasCorrln/CurrMeasCorrln/CurrMeasCorrlnPer1/CorrlnChkDEF ==
  state [ImdtCorrlnDEF,CurrMotSumDEF] = ImdtCorrlnCk(MotCurrCorrdD,MotCurrCorrdE,MotCurrCorrdF) [function]
  note: /******************************
      | Change for 2.9.0
      | CurrMotSumDEF = 0;
      | ******************************/
  state CurrMeasCorrlnNtcSet = SetNtcSts(NTCNr,ParamBit,NTCSts,NTCDebStep) [function]
  note: Rationale for CurrMotSumDEF = 0:
      | This is notifying state of health that CurrMotSum
      | is OK when it is not evaluated.   Since state of health
      | latches the most "unhealthy" value of the signal
      | it has received, this will have no impact on state of health.
  state NtcQlfr1 = GetNtcQlfrSts(NtcNr) [function]
  (default) -> (junction 141)
  (junction 141) -> (junction 150) [order 2] : {CurrMeasImdtCorrlnStsVldDEF = 1;
      | CurrMeasLongTermCorrlnStsVldDEF = 1;
      | CurrMotSumDEF = 0;}
  (junction 141) -> (junction 153) [order 1] : [SysSt == 2]
  (junction 153) -> (junction 150) [order 2] : {CurrMeasImdtCorrlnStsVldDEF = 0;
      | CurrMeasLongTermCorrlnStsVldDEF = 0;
      | CurrMotSumDEF = 0;}
  (junction 153) -> (junction 53) [order 1] : [ELECGLBPRM_IVTRCNT_CNT_U08 == 2 &&...
      |  DiagcStsIvtr2Inactv == 0 && MotCurrEolCalSt == 0]
      |
      | {[ImdtCorrlnDEF, CurrMotSumDEF] = ImdtCorrlnCk(MotCurrCorrdD, MotCurrCorrdE, MotCurrCorrdF);}
  (junction 53) -> (junction 75) [order 2]
  (junction 53) -> (junction 57) [order 1] : [ImdtCorrlnDEF == 1]
  (junction 57) -> (junction 89) : {CurrMeasImdtCorrlnStsVldDEF = 1;
      | SetNtcSts(NTCNR_0X04E, 0, 2, CurrMeasCorrlnNtc0x04EPassStep);}
  (junction 75) -> (junction 90) : {CurrMeasImdtCorrlnStsVldDEF = 0;
      | SetNtcSts(NTCNR_0X04E, 1, 3, CurrMeasCorrlnNtc0x04EFailStep);}
  (junction 89) -> (junction 93)
  (junction 90) -> (junction 93)
  (junction 93) -> (junction 102) : {CorrlnNtc4EQlfrSts = GetNtcQlfrSts(NTCNR_0X04E);}
  (junction 102) -> (junction 103) [order 1] : [CorrlnNtc4EQlfrSts == 2]
      | {CurrMeasLongTermCorrlnStsVldDEF = 0;}
  (junction 102) -> (junction 103) [order 2] : {CurrMeasLongTermCorrlnStsVldDEF = 1;}
  (junction 103) -> (junction 150)
  data: MotCurrCorrdD function_input double; MotCurrCorrdE function_input double; MotCurrCorrdF function_input double; ImdtCorrlnDEF function_output; CurrMotSumDEF function_output; NTCNr function_input; ParamBit function_input; CurrMeasCorrlnNtcSet function_output; NTCSts function_input; NTCDebStep function_input; NtcNr function_input; NtcQlfr1 function_output; MotCurrCorrdD input; MotCurrCorrdE input; MotCurrCorrdF input; CurrMeasLongTermCorrlnNtc4ESet local uint8; CorrlnCk local double; CorrlnNtc4EQlfrSts local uint8; NTC4E constant double; CurrMeasCorrlnNtc0x04EPassStep input; CurrMeasCorrlnNtc0x04EFailStep input; SysSt input; DiagcStsIvtr2Inactv input; CurrMeasImdtCorrlnStsVldDEF output uint8; CurrMeasLongTermCorrlnStsVldDEF output uint8; NTCNR_0X04E constant uint16 =78; MotCurrEolCalSt input; ELECGLBPRM_IVTRCNT_CNT_U08 input; CurrMotSumDEF output single; ImdtCorrlnDEF local double

== stateflow chart ES209A_CurrMeasCorrln/CurrMeasCorrln/CurrMeasCorrlnPer1/CorrlnChkDEF/SetNtcSts/SetNtcSts/ISO Fault Debounce Design ==
  note: Pass Loop
  note: Fail Loop
  note: 
  note: NTCSTS_PASSD           (0)
      | NTCSTS_FAILD             (1)
      | NTCSTS_PREPASSD   (2)
      | NTCSTS_PREFAILD     (3)
      |
      | SIGQLFR_NORES        (0)
      | SIGQLFR_PASSD         (1)
      | SIGQLFR_FAILD           (2)
  (default) -> (junction 89)
  (junction 89) -> (junction 95) [order 1] : [NtcSts ==3]
  (junction 89) -> (junction 93) [order 2] : [NtcSts ==2]
  (junction 89) -> (junction 141) [order 3] : [NtcSts ==1]
      | { ErrAcc = 32767;
      | Qualifier =2;
      |  }
  (junction 89) -> (junction 141) [order 4] : [NtcSts ==0]
      | { ErrAcc = -32768;
      | Qualifier=1;
      | }
  (junction 95) -> (junction 103) [order 2]
  (junction 95) -> (junction 111) [order 1] : [ErrAcc <=0]
      | {ErrAcc = DebStep;}
  (junction 93) -> (junction 123) [order 2] : {ErrAcc = ErrAcc - DebStep;}
  (junction 93) -> (junction 123) [order 1] : [(ErrAcc - DebStep) <= -32768]
      | { ErrAcc = -32768;
      | Qualifier=1;}
  (junction 103) -> (junction 111) [order 1] : [(ErrAcc + DebStep) <32767]
      | {ErrAcc = ErrAcc + DebStep;}
  (junction 103) -> (junction 111) [order 2] : {ErrAcc = 32767;
      | Qualifier = 2;}
  (junction 123) -> (junction 141)
  (junction 111) -> (junction 141)
  (junction 141) -> (junction 159) [order 1] : [SvcClr ==1]
      | {ErrAcc = 0;
      | Qualifier =0;}
  (junction 141) -> (junction 159) [order 2]
  data: NtcSts input uint8; Qualifier output uint8; DebStep input int32; ErrAcc output single; SvcClr input

== stateflow chart ES209A_CurrMeasCorrln/CurrMeasCorrln/CurrMeasCorrlnPer1/Signal Availability/Signal Availability Check En/SigAvlChk1/SigAvlChkRev2 ==
  note: SigAvl
      | False = 0
      | Pass = 1
  note: SigQlfr
      | 0 = No Result
      | 1 = Pass
      | 2 = Fail
  (default) -> (junction 109)
  (junction 109) -> (junction 121) [order 1] : [SigRollgCnt ==LstRollgCnt]
  (junction 121) -> (junction 125) [order 2] : {
      | StallCntOutp = LstStallCnt +1;
      | }
  (junction 109) -> (junction 127) [order 2]
  (junction 121) -> (junction 125) [order 1] : [LstStallCnt == 255]
      | {
      | StallCntOutp = 255;
      | }
  (junction 127) -> (junction 125) : {
      | StallCntOutp = 0;
      | }
  (junction 125) -> (junction 126)
  (junction 126) -> (junction 123) [order 1] : [StallCntOutp >=kMaxStallCnt]
  (junction 126) -> (junction 105) [order 2]
  (junction 105) -> (junction 123) [order 2]
  (junction 105) -> (junction 117) [order 1] : [SigQlfr<2]
  (junction 123) -> (junction 111) : {
      | SigAvl =0;
      | }
  (junction 117) -> (junction 111) : {
      | SigAvl = 1;
      | }
  data: SigRollgCnt input; SigQlfr input; kMaxStallCnt input; SigAvl output uint8; LstRollgCnt input uint8; LstStallCnt input uint8; StallCntOutp output uint8

== stateflow chart ES209A_CurrMeasCorrln/CurrMeasCorrln/CurrMeasCorrlnPer1/Signal Availability/Signal Availability Check En/SigAvlChk2/SigAvlChkRev2 ==
  note: SigAvl
      | False = 0
      | Pass = 1
  note: SigQlfr
      | 0 = No Result
      | 1 = Pass
      | 2 = Fail
  (default) -> (junction 123)
  (junction 123) -> (junction 135) [order 1] : [SigRollgCnt ==LstRollgCnt]
  (junction 135) -> (junction 139) [order 2] : {
      | StallCntOutp = LstStallCnt +1;
      | }
  (junction 123) -> (junction 141) [order 2]
  (junction 135) -> (junction 139) [order 1] : [LstStallCnt == 255]
      | {
      | StallCntOutp = 255;
      | }
  (junction 141) -> (junction 139) : {
      | StallCntOutp = 0;
      | }
  (junction 139) -> (junction 140)
  (junction 140) -> (junction 136) [order 1] : [StallCntOutp >=kMaxStallCnt]
  (junction 140) -> (junction 119) [order 2]
  (junction 136) -> (junction 137)
  (junction 119) -> (junction 137) [order 2]
  (junction 119) -> (junction 131) [order 1] : [SigQlfr<2]
  (junction 137) -> (junction 125) : {
      | SigAvl =0;
      | }
  (junction 131) -> (junction 125) : {
      | SigAvl = 1;
      | }
  data: SigRollgCnt input; SigQlfr input; kMaxStallCnt input; SigAvl output uint8; LstRollgCnt input uint8; LstStallCnt input uint8; StallCntOutp output uint8
